simulink model "task1_simple_model_withdelay"  (R2020b)
settings: Solver=VariableStepAuto  StartTime=0.0  StopTime=60  RelTol=1e-3
libraries: simulink x5, dspsigops x4
settings Model: Creator=Isabel  LastModifiedBy=Isabel

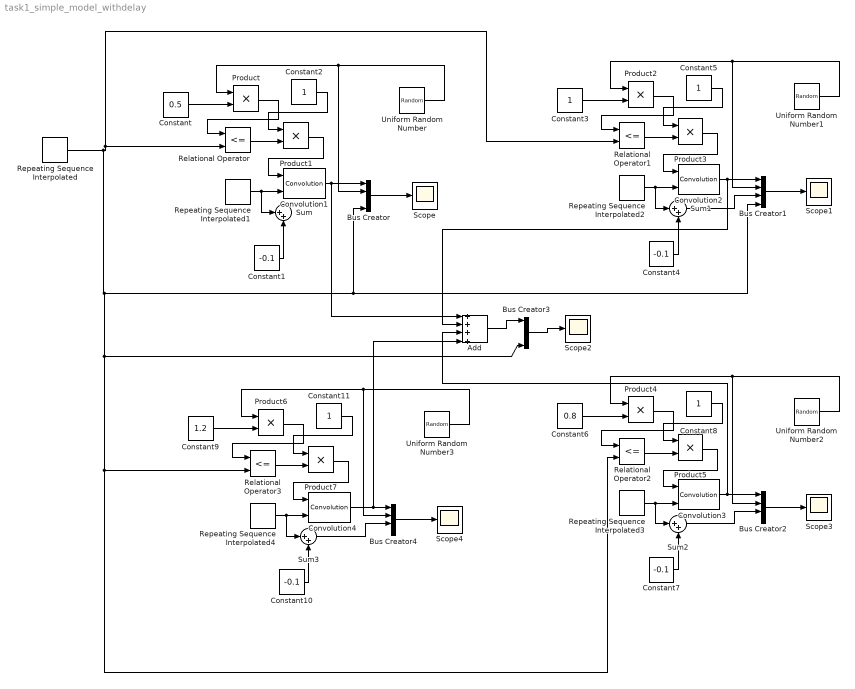
== system task1_simple_model_withdelay ==
  Add : Sum  Inputs=++++
  Bus Creator{,1..4} (5 alike) : BusCreator  Inputs=4
  Constant : Constant  Value=0.5
  Constant{1,4,7,10} (4 alike) : Constant  Value=-0.1
  Constant{2..3,5,8,11} (5 alike) : Constant
  Constant6 : Constant  Value=0.8
  Constant9 : Constant  Value=1.2
  Convolution{1..4} (4 alike) : dspsigops/Convolution  domain=Time  roundingMode=Floor  overflowMode=off  outputDataTypeStr=Inherit: Same as accumulator  outputMin=[]  outputMax=[]  outputLastDataTypeStr=Inherit: Same as accumulator
      settings: SourceProductBaseCode=DS
  Product{,1..7} (8 alike) : Product
  Relational Operator{,1..3} (4 alike) : RelationalOperator  Operator=<=  OutDataTypeStr=boolean  RndMeth=Simplest
  Repeating Sequence Interpolated : simulink/Sources/Repeating Sequence Interpolated  OutValues=[0 0.027 0.15 0.364 0.49 0.52 0.513 0.489 0.277 0.233 0.18 0.074 0.0177 0 0].'  TimeValues=[0 0.7 1.2 1.6 1.9 2.1 2.2 2.3 2.9 3.1 3.5 4.4 5.2 6.4 8].'  LookUpMeth=Interpolation-Use End Values  tsamp=0.1  OutMin=[]  OutMax=[]  OutDataTypeStr=double  OutputDataTypeScalingMode=double  OutDataType=fixdt(0,8)  OutScaling=2^-10
  Repeating Sequence Interpolated{1..4} (4 alike) : simulink/Sources/Repeating Sequence Interpolated  OutValues=[0.005 0.01 0.018 0.021 0.033 0.053 0.048 0.028 0.01 0.002 0 0].'  TimeValues=[0 0.0015 0.0035 0.004 0.006 0.01 0.014 0.018 0.02 0.026 0.033 0.05].'  LookUpMeth=Interpolation-Use End Values  tsamp=0.0005  OutMin=[]  OutMax=[]  OutDataTypeStr=double  OutputDataTypeScalingMode=double  OutDataType=fixdt(0,8)  OutScaling=2^-10
  Scope{,1..4} (5 alike) : Scope
  Sum{,1..3} (4 alike) : Sum  Inputs=|++
  Uniform Random Number : UniformRandomNumber  Minimum=0  SampleTime=0.1
  Uniform Random Number1 : UniformRandomNumber  Minimum=0  Seed=3  SampleTime=0.1
  Uniform Random Number2 : UniformRandomNumber  Minimum=0  Seed=8  SampleTime=0.1
  Uniform Random Number3 : UniformRandomNumber  Minimum=0  Seed=20  SampleTime=0.1
  wires:
  Uniform Random Number/1 -> Bus Creator/2, Product/1
  Product/1 -> Relational Operator/1
  Bus Creator/1 -> Scope/1
  Convolution1/1 -> Add/1, Bus Creator/1
  Repeating Sequence Interpolated1/1 -> Sum/1, Convolution1/2
  Relational Operator/1 -> Product1/2
  Product1/1 -> Convolution1/1
  Constant2/1 -> Product1/1
  Constant/1 -> Product/2
  Constant1/1 -> Sum/2
  Repeating Sequence Interpolated/1 -> Bus Creator3/4, Relational Operator3/2, Relational Operator2/2, Bus Creator/4, Bus Creator1/4, Relational Operator/2, Relational Operator1/2
  Constant5/1 -> Product3/1
  Sum1/1 -> Bus Creator1/3
  Product3/1 -> Convolution2/1
  Constant4/1 -> Sum1/2
  Relational Operator1/1 -> Product3/2
  Constant3/1 -> Product2/2
  Bus Creator1/1 -> Scope1/1
  Product2/1 -> Relational Operator1/1
  Repeating Sequence Interpolated2/1 -> Sum1/1, Convolution2/2
  Convolution2/1 -> Add/2, Bus Creator1/1
  Uniform Random Number1/1 -> Bus Creator1/2, Product2/1
  Uniform Random Number2/1 -> Bus Creator2/2, Product4/1
  Repeating Sequence Interpolated3/1 -> Sum2/1, Convolution3/2
  Convolution3/1 -> Add/3, Bus Creator2/1
  Product4/1 -> Relational Operator2/1
  Bus Creator2/1 -> Scope3/1
  Constant6/1 -> Product4/2
  Product5/1 -> Convolution3/1
  Relational Operator2/1 -> Product5/2
  Sum2/1 -> Bus Creator2/3
  Constant8/1 -> Product5/1
  Constant7/1 -> Sum2/2
  Add/1 -> Bus Creator3/1
  Bus Creator3/1 -> Scope2/1
  Constant11/1 -> Product7/1
  Constant9/1 -> Product6/2
  Constant10/1 -> Sum3/2
  Sum3/1 -> Bus Creator4/3
  Product7/1 -> Convolution4/1
  Convolution4/1 -> Add/4, Bus Creator4/1
  Relational Operator3/1 -> Product7/2
  Product6/1 -> Relational Operator3/1
  Uniform Random Number3/1 -> Bus Creator4/2, Product6/1
  Repeating Sequence Interpolated4/1 -> Sum3/1, Convolution4/2
  Bus Creator4/1 -> Scope4/1
